simulink model "com_FT60_2020a"  (R2020a)
settings: Solver=FixedStepAuto  StartTime=0.0  StopTime=180  RelTol=1e-3  EnableMultiTasking=on
values from neighbouring files (symbols this model uses):
  node = scgtnodestruct(node)    [initializeSCRAMNetGT.m]    (also in initializeSCRAMNetGT_com.m)
libraries: speedgoatlib_IO901_IO902 x3, slrtlib x2
settings Model: SimulationMode=external  Creator=C086922  LastModifiedBy=C086922
settings SolverCC: ConcurrentTasks=on  AutoInsertRateTranBlk=on
settings DataIOCC: SaveFormat=StructureWithTime
settings OptimizationCC: BlockReduction=off  OptimizeBlockIOStorage=off
settings HardwareCC: ProdBitPerPointer=32  ProdBitPerSizeT=32  ProdBitPerPtrDiffT=32  ProdLargestAtomicFloat=None  ProdWordSize=32  ProdLongLongMode=on  ProdHWDeviceType=Generic->32-bit x86 compatible
settings RTWCC: Description=Simulink Real-Time  SystemTargetFile=slrt.tlc  TemplateMakefile=slrt_default_tmf  CodeExecutionProfiling=on  RTWCompilerOptimization=on
settings SimulinkRealTimeCC: SupportVariableSizeSignals=on  RL32LogTETModifier=off  xPCConcurrentTasks=on

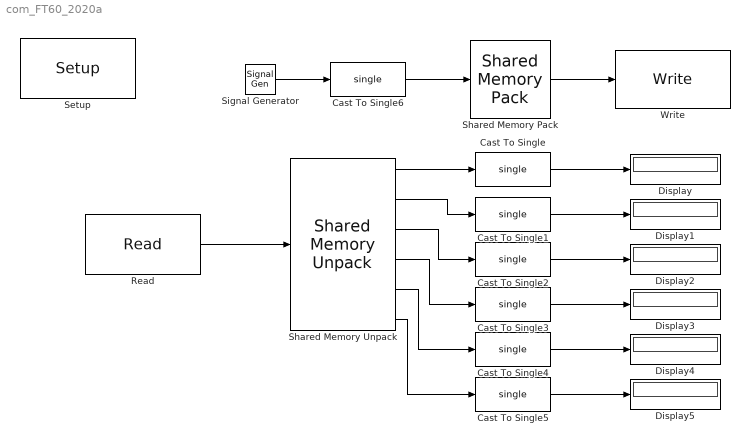
== system com_FT60_2020a ==
  Cast To Single{,1..6} (7 alike) : DataTypeConversion  OutDataTypeStr=single
  Display{,1..5} (6 alike) : Display
  "Read " : speedgoatlib_IO901_IO902/Read   id=1  partition=node.Partitions(8:13)  ts=0.001  pci=-1
      settings: SourceProductName=Simulink Real-Time: Speedgoat I/O Blockset
  "Setup " : speedgoatlib_IO901_IO902/Setup   id=1  node=node  pci=-1
      settings: SourceProductName=Simulink Real-Time: Speedgoat I/O Blockset
  "Shared Memory Pack " : slrtlib/Shared Memory/Shared Memory Pack   partition=node.Partitions(3)
      settings: SourceProductBaseCode=XP
  "Shared Memory Unpack " : slrtlib/Shared Memory/Shared Memory Unpack   partition=node.Partitions(8:13)
      settings: SourceProductBaseCode=XP
  Signal Generator : SignalGenerator  Amplitude=0.5  Frequency=0.1  Units=rad/sec
  "Write " : speedgoatlib_IO901_IO902/Write   id=1  partition=node.Partitions(3)  ts=0.001  pci=-1
      settings: SourceProductName=Simulink Real-Time: Speedgoat I/O Blockset
  wires:
  "Read "/1 -> "Shared Memory Unpack "/1
  "Shared Memory Unpack "/1 -> Cast To Single/1
  "Shared Memory Unpack "/2 -> Cast To Single1/1
  "Shared Memory Unpack "/3 -> Cast To Single2/1
  "Shared Memory Unpack "/4 -> Cast To Single3/1
  "Shared Memory Unpack "/5 -> Cast To Single4/1
  "Shared Memory Unpack "/6 -> Cast To Single5/1
  Cast To Single/1 -> Display/1
  Cast To Single1/1 -> Display1/1
  Cast To Single2/1 -> Display2/1
  Cast To Single3/1 -> Display3/1
  Cast To Single4/1 -> Display4/1
  Cast To Single5/1 -> Display5/1
  "Shared Memory Pack "/1 -> "Write "/1
  Cast To Single6/1 -> "Shared Memory Pack "/1
  Signal Generator/1 -> Cast To Single6/1
